simulink model "main_RI_LIEKF_GNSSOutrage"  (R2023a)
settings: Solver=FixedStepAuto  StartTime=0.0  StopTime=220  FixedStep=0.01  RelTol=1e-3
InitFcn:
  | initNavigation0612_AOA;
values from neighbouring files (symbols this model uses):
  CF_enable = 0    [initNavigation.m]
  dt = 0.01    [initNavigation.m]
  dtDelay = -0.03    [initNavigation.m]
  g0 = 9.795    [initNavigation.m]
  gam0_rad = 0/57.3    (= 0)    [initNavigation.m]
  GNSSoutragetime = 90    [initNavigation.m]
  H_sensor_type = 0    [initNavigation.m]
  KF_enable = 1    [initNavigation.m]
  P0 = diag([1*ones(3,1);0.01*ones(3,1);0.1*ones(3,1);0.001*ones(3,1);0.00001*ones(3,1)])    [initNavigation.m]
  P0_RIEKF = diag([1*ones(3,1);0.01*ones(3,1);0.1*ones(3,1);0.001*ones(3,1);0.00001*ones(3,1);      0.01*ones(3,1);[0;2;2]/57.3;[0.1;0.1;0.1]])^2    [initNavigation.m]
  pd0 = 0    [initNavigation.m]
  pe0 = 0    [initNavigation.m]
  phi0_rad = 0/57.3    (= 0)    [initNavigation.m]
  pn0 = 0    [initNavigation.m]
  psi = -178    [initNavigation.m]
  psi0_rad = 0/57.3    (= 0)    [initNavigation.m]
  state_dim = 24    [initNavigation.m]
  Time = 0:0.01:(size(traindata.AttackAngle,1) - 1)*0.01    [NNLiftCoefficientFit.m]
  vd0 = 0    [initNavigation.m]
  ve0 = 0    [initNavigation.m]
  vn0 = 0    [initNavigation.m]
undefined symbols (not defined in the file or in its folder): DiscIntNeverNeededParam, Discrete, INS_CONST, INS_EXPORT, INS_PARAM, magnitude, p, param, pInitialization, sys
libraries: simulink_extras x94, simulink x82, dspstat3 x70, sharedtransform x60, ctrlSharedLib x36, sharedTrackingLibrary x22, matrix_library x15, FMT_Model_Lib x13, deeplib x8, dspsolvers x4, vrlib x4, aerolibconvert2 x1
(part 3 of 28)

== system main_RI_LIEKF_GNSSOutrage/State estimation/15dim KF1/Error State Kalman Filter ==
  Sensor_data : Inport
  INS state : Inport  Port=2
  Add : Sum  Inputs=+-
  Bus Creator : BusCreator  Inputs=5
  Bus Selector : BusSelector  OutputSignals=QGC_sensor_reinit,GPS_Data.pos_N_gps,GPS_Data.pos_E_gps,GPS_Data.pos_D_gps,GPS_Data.vn_gps,GPS_Data.ve_gps,GPS_Data.vd_gps,vicon.vicon_posxyz,QGC_sensor_reinit
  Bus Selector2 : BusSelector  OutputSignals=RotationData.DCM_b_n,INSstate_v,INSstste_p,INSstate_w,INSstate_fb
  Cal Phi : Subsystem
  Cal Q : Subsystem
  Constant6 : Constant  Value=[eye(3),zeros(3,12)]  OutDataTypeStr=single
  Constant7 : Constant  Value=zeros(15,1)  OutDataTypeStr=single
  Data Store Read1 : DataStoreRead  DataStoreName=feedback_flag  IndexOptions=Index vector (dialog)  Indices=1  OutputSizes=1
  Data Store Read2 : DataStoreRead  DataStoreName=feedback_flag  IndexOptions=Index vector (dialog)  Indices=1  OutputSizes=1
  Data Type Conversion{1..3,5} (4 alike) : DataTypeConversion  OutDataTypeStr=single  SaturateOnIntegerOverflow=off  RndMeth=Floor
  Extract Diagonal : matrix_library/Extract Diagonal
  GNSS/INS Kalman Filter1 : Subsystem  AncestorBlock=ctrlSharedLib/Kalman Filter  mask(ctrlKalmanFilter){TimeDomain=Discrete-Time, UseCurrentEstimator=off, ModelSource=Input port, ModelSourceVariable=sys, A=0.95*eye(2), B=eye(2), C=eye(2), D=zeros(2), NumberOfStates=15, NumberOfInputs=0, NumberOfOutputs=3, InitialEstimateSource=Input port, X0=0, P0=10, UseK=off, UseGH=off, NumberOfProcessNoiseInputs=2, G=diag([zeros(3,1);ones(12,1)]), TimeInvariantG=off, H=0, TimeInvariantH=on, Q=diag([zeros(3,1);1e-2*ones(3,1);1e-4*ones(3,1);zeros(3,1);1e-5*ones(3,1)]), TimeInvariantQ=off, R=diag([0.001,0.001,0.001]), TimeInvariantR=on, N=0, TimeInvariantN=on, AddInputPort=off, AddEnablePort=on, ExternalReset=Rising, OutputEstimatedY=off, OutputP=on, Ts=dt}
      mask prompts: TimeDomain "Controllib:blocks:maskPromptKFTimeDomain"; UseCurrentEstimator "Controllib:blocks:maskPromptKFUseCurrentMeasurement"; ModelSource "Controllib:blocks:maskPromptKFModelSource"; ModelSourceVariable "Controllib:blocks:maskPromptKFModelSourceVariable"; A "Controllib:blocks:maskPromptKFA"; B "Controllib:blocks:maskPromptKFB"; C "Controllib:blocks:maskPromptKFC"; D "Controllib:blocks:maskPromptKFD"; NumberOfStates "Controllib:blocks:maskPromptKFNumberOfStates"; NumberOfInputs "Controllib:blocks:maskPromptKFNumberOfInputs"; NumberOfOutputs "Controllib:blocks:maskPromptKFNumberOfOutputs"; InitialEstimateSource "Controllib:blocks:maskPromptKFSource"; X0 "Controllib:blocks:maskPromptKFX0DT"; P0 "Controllib:blocks:maskPromptKFP0DT"; UseK "Controllib:blocks:maskPromptKFUseK"; UseGH "Controllib:blocks:maskPromptKFUseGH"; NumberOfProcessNoiseInputs "Controllib:blocks:maskPromptKFNumberOfProcessNoiseInputs"; G "Controllib:blocks:maskPromptKFG"; TimeInvariantG "Controllib:blocks:maskPromptKFTimeInvariantG"; H "Controllib:blocks:maskPromptKFH"; TimeInvariantH "Controllib:blocks:maskPromptKFTimeInvariantH"; Q "Controllib:blocks:maskPromptKFQ"; TimeInvariantQ "Controllib:blocks:maskPromptKFTimeInvariantQ"; R "Controllib:blocks:maskPromptKFR"; TimeInvariantR "Controllib:blocks:maskPromptKFTimeInvariantR"; N "Controllib:blocks:maskPromptKFN"; TimeInvariantN "Controllib:blocks:maskPromptKFTimeInvariantN"; AddInputPort "Controllib:blocks:maskPromptKFAddInputPort"; AddEnablePort "Controllib:blocks:maskPromptKFAddEnablePort"; ExternalReset "Simulink:blkprm_prompts:DelayBlkExternalReset"; OutputEstimatedY "Controllib:blocks:maskPromptKFOutputEstimatedY"; OutputP "Controllib:blocks:maskPromptKFOutputP"; Ts "Controllib:blocks:maskPromptKFTs"
      mask help: Controllib:blocks:maskPromptKFDescription
      mask init:
      | dlgParams.TimeDomain = TimeDomain;
      | dlgParams.UseCurrentEstimator = UseCurrentEstimator;
      | dlgParams.ModelSource = ModelSource;
      | dlgParams.ModelSourceVariable = ModelSourceVariable;
      | dlgParams.A = A;
      | dlgParams.B = B;
      | dlgParams.C = C;
      | dlgParams.D = D;
      | dlgParams.ModelHasFeedthrough = true();
      | dlgParams.NumberOfStates = NumberOfStates;
      | dlgParams.NumberOfInputs = NumberOfInputs;
      | dlgParams.NumberOfOutputs = NumberOfOutputs;
      | dlgParams.InitialEstimateSource = InitialEstimateSource;
      | dlgParams.X0 = X0;
      | dlgParams.P0 = P0;
      | dlgParams.UseGH = UseGH;
      | dlgParams.UseK = UseK;
      | dlgParams.NumberOfProcessNoiseInputs = NumberOfProcessNoiseInputs;
      | dlgParams.G = G;
      | dlgParams.TimeInvariantG = TimeInvariantG;
      | dlgParams.H = H;
      | dlgParams.TimeInvariantH = TimeInvariantH;
      | dlgParams.Q = Q;
      | dlgParams.TimeInvariantQ = TimeInvariantQ;
      | dlgParams.R = R;
      | dlgParams.TimeInvariantR = TimeInvariantR;
      | dlgParams.N = N;
      | dlgParams.TimeInvariantN = TimeInvariantN;
      | % Block options panel
      | dlgParams.OutputEstimatedY = OutputEstimatedY;
      | dlgParams.OutputP = OutputP;
      | dlgParams.AddEnablePort = AddEnablePort;
      | dlgParams.AddInputPort = AddInputPort;
      | dlgParams.ExternalReset = ExternalReset;
      | dlgParams.Ts = Ts;
      | [pInitialization,p] = ...
      |     controllib.internal.blocks.kalmanfilter.maskInitializationFcn(gcbh,dlgParams);
      | % Avoid storing dlg variables twice in the MaskWSVariables 
      | % block property
      | clear dlgParams;
      settings: LibrarySourceBlock=ctrlSharedLib/Kalman Filter
      mask Help: eval('controllib.internal.blocks.kalmanfilter.launchDocPage()')
      mask TypeOptions TimeDomain: Controllib:blocks:maskPromptKFTimeDomainDT | Controllib:blocks:maskPromptKFTimeDomainCT
      mask Callback TimeDomain: controllib.internal.blocks.kalmanfilter.dialogCallbacks(gcbh(),'comboBoxTimeDomain');
      mask Callback UseCurrentEstimator: controllib.internal.blocks.kalmanfilter.dialogCallbacks(gcbh(),'checkBoxUseCurrentEstimator');
      mask TypeOptions ModelSource: Controllib:blocks:maskPromptKFModelSourceLTIObject | Controllib:blocks:maskPromptKFModelSourceMatrices | Controllib:blocks:maskPromptKFSourceInport
      mask Callback ModelSource: controllib.internal.blocks.kalmanfilter.dialogCallbacks(gcbh(),'comboBoxModelSource');
      mask Callback ModelSourceVariable: controllib.internal.blocks.kalmanfilter.dialogCallbacks(gcbh(),'editBoxModelSourceVariable')
      mask TypeOptions InitialEstimateSource: Controllib:blocks:maskPromptKFSourceDialog | Controllib:blocks:maskPromptKFSourceInport
      mask Callback InitialEstimateSource: controllib.internal.blocks.kalmanfilter.dialogCallbacks(gcbh(),'comboBoxInitialEstimateSource');
      mask Callback UseK: controllib.internal.blocks.kalmanfilter.dialogCallbacks(gcbh(),'checkBoxUseK');
      mask Callback UseGH: controllib.internal.blocks.kalmanfilter.dialogCallbacks(gcbh(),'checkBoxUseGH');
      mask Callback TimeInvariantG: controllib.internal.blocks.kalmanfilter.dialogCallbacks(gcbh(),'checkBoxTimeInvariantGH');
      mask Callback TimeInvariantH: controllib.internal.blocks.kalmanfilter.dialogCallbacks(gcbh(),'checkBoxTimeInvariantGH');
      mask Callback TimeInvariantQ: controllib.internal.blocks.kalmanfilter.dialogCallbacks(gcbh(),'checkBoxTimeInvariantQRN');
      mask Callback TimeInvariantR: controllib.internal.blocks.kalmanfilter.dialogCallbacks(gcbh(),'checkBoxTimeInvariantQRN');
      mask Callback TimeInvariantN: controllib.internal.blocks.kalmanfilter.dialogCallbacks(gcbh(),'checkBoxTimeInvariantQRN');
      mask Callback AddInputPort: controllib.internal.blocks.kalmanfilter.dialogCallbacks(gcbh(),'checkBoxAddInputPort');
      mask TypeOptions ExternalReset: MemoryX/ExternalReset
      mask Callback OutputP: controllib.internal.blocks.kalmanfilter.dialogCallbacks(gcbh(),'checkBoxOutputP');
      mask DialogControl DescGroupVar Prompt: Controllib:blocks:maskPromptKFTitle
      mask DialogControl FilterSettingsContainer Prompt: Controllib:blocks:maskPromptKFContainerFilterSettings
      mask DialogControl TimeDomain Prompt: 时域:
      mask DialogControl UseCurrentEstimator Prompt: 使用当前测量 y[n] 来改进 xhat[n]
      mask DialogControl ModelParameterContainer Prompt: Controllib:blocks:maskPromptKFTabModelParameters
      mask DialogControl SystemModelContainer Prompt: Controllib:blocks:maskPromptKFContainerSystemModel
      mask DialogControl ModelSource Prompt: 模型源:
      mask DialogControl ModelSourceVariable Prompt: 变量:
      mask DialogControl A Prompt: A:
      mask DialogControl B Prompt: B:
      mask DialogControl C Prompt: C:
      mask DialogControl D Prompt: D:
      mask DialogControl NumberOfStates Prompt: 状态数量:
      mask DialogControl NumberOfInputs Prompt: 输入数目:
      mask DialogControl NumberOfOutputs Prompt: 输出数目:
      mask DialogControl InitialEstimatesContainer Prompt: Controllib:blocks:maskPromptKFContainerInitialEstimates
      mask DialogControl InitialEstimateSource Prompt: 源:
      mask DialogControl X0 Prompt: 初始状态 x[0]:
      mask DialogControl P0 Prompt: 状态估计误差协方差 P[0]
      mask DialogControl NoiseCharacteristicsContainer Prompt: Controllib:blocks:maskPromptKFContainerNoiseCharacteristics
      mask DialogControl UseK Prompt: 使用来自模型变量的 Kalman 增益 K
      mask DialogControl UseGH Prompt: 使用 G 和 H 矩阵(默认 G=I，H=0)
      mask DialogControl NumberOfProcessNoiseInputs Prompt: 过程噪声输入数目:
      mask DialogControl G Prompt: G:
      mask DialogControl TimeInvariantG Prompt: 时不变 G
      mask DialogControl H Prompt: H:
      mask DialogControl TimeInvariantH Prompt: 时不变 H
      mask DialogControl Q Prompt: Q:
      mask DialogControl TimeInvariantQ Prompt: 时不变 Q
      mask DialogControl R Prompt: R:
      mask DialogControl TimeInvariantR Prompt: 时不变 R
      mask DialogControl N Prompt: N:
      mask DialogControl TimeInvariantN Prompt: 时不变 N
      mask DialogControl OptionsContainer Prompt: Controllib:blocks:maskPromptKFTabOptions
      mask DialogControl AdditionalInportsContainer Prompt: Controllib:blocks:maskPromptKFContainerAdditionalInports
      mask DialogControl AddInputPort Prompt: 添加输入端口 u
      mask DialogControl AddEnablePort Prompt: 添加输入端口 Enable 以控制测量更新
      mask DialogControl ExternalReset Prompt: 外部重置:
      mask DialogControl AdditionalOutportsContainer Prompt: Controllib:blocks:maskPromptKFContainerAdditionalOutports
      mask DialogControl OutputEstimatedY Prompt: 输出估计的模型输出 y
      mask DialogControl OutputP Prompt: 输出状态估计误差协方差 P
      mask DialogControl Ts Prompt: 采样时间(-1 表示继承):
  Logical Operator : Logic  Commented=on  Operator=OR  AllPortsSameDT=off  OutDataTypeStr=boolean
  MATLAB Function : MATLAB Function  TreatAsAtomicUnit=on
  MATLAB Function2 : MATLAB Function  TreatAsAtomicUnit=on
  Memory : Memory
  Mux : Mux  Inputs=3
  Mux1 : Mux  Inputs=3
  Rate Transition : RateTransition  OutPortSampleTime=dt
  Rate Transition1 : RateTransition
  Rate Transition2 : RateTransition  OutPortSampleTime=dt
  Rate Transition3 : RateTransition  OutPortSampleTime=dt
  Scope{,2..3,5,7,9..10} (7 alike) : Scope
  Subsystem : Subsystem
  Terminator : Terminator
  delta_state : Outport
  Measuemrnt Enable Flag : Outport  Port=2
  covariance : Outport  Port=3
  wires:
  Data Store Read2/1 -> Logical Operator/1, GNSS/INS Kalman Filter1/5(Reset)
  Bus Selector/9 -> [QGC_init]  "<QGC_sensor_reinit>"
  Mux/1 -> [pos_NED]
  Rate Transition3/1 -> GNSS/INS Kalman Filter1/4(Enable)
  [Enable] -> Rate Transition3/1
  Memory/1 -> MATLAB Function/1(u)
  Bus Creator/1 -> delta_state/1
  MATLAB Function/3(dtheta) -> Bus Creator/3  "KFState_dtheta"
  Data Type Conversion1/1 -> Memory/1
  MATLAB Function/1(dp) -> Bus Creator/1  "KFState_dp"
  MATLAB Function/5(dg) -> Bus Creator/5  "KFState_da"
  MATLAB Function/2(dv) -> Bus Creator/2  "KFState_dv"
  MATLAB Function/4(da) -> Bus Creator/4  "KFState_da"
  Bus Selector2/3 -> [p_INS]  "<INSstste_p>"
  Bus Selector2/1 -> [DCM_b_n]  "<DCM_b_n>"
  Bus Selector2/5 -> [fbxyz]  "<INSstate_fb>"
  Bus Selector2/4 -> [wxyz]  "<INSstate_w>"
  INS state/1 -> Bus Selector2/1
  [Enable] -> Measuemrnt Enable Flag/1
  Bus Selector/4 -> Mux/3  "<pos_D_gps>"
  Bus Selector/2 -> Mux/1  "<pos_N_gps>"
  Bus Selector/3 -> Mux/2  "<pos_E_gps>"
  Bus Selector/7 -> Mux1/3  "<vd_gps>"
  Bus Selector/5 -> Mux1/1  "<vn_gps>"
  Mux1/1 -> Scope2/1, Terminator/1
  Sensor_data/1 -> Bus Selector/1
  Bus Selector/6 -> Mux1/2  "<ve_gps>"
  Extract Diagonal/1 -> Scope9/1, covariance/1
  GNSS/INS Kalman Filter1/2(P) -> Extract Diagonal/1
  Data Store Read1/1 -> Scope7/1
  Rate Transition2/1 -> Data Type Conversion5/1
  Cal Q/1(Qd) -> Rate Transition2/1
  MATLAB Function2/1(P) -> Data Type Conversion2/1
  Data Type Conversion5/1 -> GNSS/INS Kalman Filter1/8(Q)
  Cal Phi/1(Phi) -> Rate Transition1/1
  [DCM_b_n] -> Cal Phi/1(<DCM_b_n>)
  [pos_NED] -> Subsystem/1(data)
  [fbxyz] -> Cal Phi/3(axyz)
  Data Type Conversion2/1 -> GNSS/INS Kalman Filter1/3(P0)
  [pos_NED] -> Add/2, Scope3/1
  [p_INS] -> Add/1
  Rate Transition1/1 -> Data Type Conversion3/1
  [DCM_b_n] -> Cal Q/1(<DCM_b_n>)
  [wxyz] -> Cal Phi/2(wxyz)
  Add/1 -> Rate Transition/1, Scope10/1
  Data Type Conversion3/1 -> GNSS/INS Kalman Filter1/6(A)
  Constant6/1 -> GNSS/INS Kalman Filter1/7(C)
  [wxyz] -> Cal Q/2(wxyz)
  Rate Transition/1 -> GNSS/INS Kalman Filter1/1(y)
  Subsystem/1(flag) -> [Enable], Scope5/1
  GNSS/INS Kalman Filter1/1(xhat) -> Data Type Conversion1/1, Scope/1
  Constant7/1 -> GNSS/INS Kalman Filter1/2(X0)

== system main_RI_LIEKF_GNSSOutrage/State estimation/15dim KF1/INS propogation ==
  note: q(1:3)
  Sensor_data : Inport
  Measuemrnt Enable Flag : Inport  Port=2
  delta_state : Inport  Port=3
  Bus Creator : BusCreator  Inputs=7
  Bus Selector : BusSelector  OutputSignals=IMU_Data.gyro_B_rad/s_LPF,IMU_Data.accl_B_m/s2_LPF,MAGN_Data,QGC_sensor_reinit,GPS_Data.pos_N_gps,GPS_Data.pos_E_gps,GPS_Data.pos_D_gps,GPS_Data.vn_gps,GPS_Data.ve_gps,GPS_Data.vd_gps,vicon.vicon_posxyz
  Bus Selector1 : BusSelector  OutputSignals=DCM_b_n
  Bus Selector2 : BusSelector  OutputSignals=KFState_dp (signal 1),KFState_dv (signal 2),KFState_dtheta (signal 3),KFState_da (signal 4),KFState_da (signal 5)
  Data Type Conversion : DataTypeConversion  OutDataTypeStr=single  SaturateOnIntegerOverflow=off  RndMeth=Floor
  Init_PVQ2 : Subsystem
  Mux : Mux  Inputs=3
  Mux1 : Mux  Inputs=3
  accl bias compensation : Subsystem
  att_update : Subsystem
  gyro bias compensation : Subsystem
  vel_pos_update : Subsystem
  INSstate : Outport
  wires:
  Mux/1 -> [pos_NED]
  Bus Selector/2 -> [accl_raw]  "<accl_B_m/s2_LPF>"
  [accl_raw] -> accl bias compensation/1(raw <accl_B_m/s2_LPF>)
  [gyro_raw] -> gyro bias compensation/1(raw <gyro_B_rad/s_LPF>)
  Bus Selector2/5 -> [ddg]  "<KFState_da (signal 5)>"
  Bus Selector2/4 -> [dda]  "<KFState_da (signal 4)>"
  Bus Selector2/3 -> [dtheta]  "<KFState_dtheta (signal 3)>"
  Bus Selector2/2 -> [dv]  "<KFState_dv (signal 2)>"
  Bus Selector2/1 -> [dp]  "<KFState_dp (signal 1)>"
  delta_state/1 -> Bus Selector2/1
  [da] -> Bus Creator/7  "INSstate_da"
  [dg] -> Bus Creator/6  "INSstate_dg"
  gyro bias compensation/2(dg) -> [dg]
  gyro bias compensation/1(wb) -> [wxyz]
  Measuemrnt Enable Flag/1 -> gyro bias compensation/3(Measuemrnt Enable Flag)
  [ddg] -> gyro bias compensation/2(ddg)
  accl bias compensation/2(da) -> [da]
  accl bias compensation/1(fb) -> [fbxyz]
  [dda] -> accl bias compensation/2(dda)
  Bus Creator/1 -> INSstate/1
  att_update/1(att_update) -> Bus Creator/1, Bus Selector1/1  "RotationData"
  [fbxyz] -> Bus Creator/5  "INSstate_fb"
  [wxyz] -> Bus Creator/4  "INSstate_w"
  vel_pos_update/1(p_k) -> Bus Creator/2  "INSstste_p"
  [QGC_init] -> Init_PVQ2/1(QGC_sensor_reinit)
  [dv] -> vel_pos_update/7(dv)
  vel_pos_update/2(V) -> Bus Creator/3  "INSstate_v"
  Bus Selector1/1 -> vel_pos_update/1(<DCM_b_n>)  "<DCM_b_n>"
  Bus Selector/1 -> [gyro_raw]  "<gyro_B_rad/s_LPF>"
  Bus Selector/4 -> [QGC_init]  "<QGC_sensor_reinit>"
  [Magn] -> Init_PVQ2/3(Magn_B_guess_LPF)
  [dp] -> vel_pos_update/6(dp)
  Data Type Conversion/1 -> Init_PVQ2/5(vel_NED)
  [pos_NED] -> Init_PVQ2/4(pos_NED)
  [QGC_init] -> vel_pos_update/5(QGC_init)
  Bus Selector/9 -> Mux1/2  "<ve_gps>"
  Init_PVQ2/3(p0) -> vel_pos_update/4(p0)
  Init_PVQ2/2(v0) -> vel_pos_update/3(v0)
  [fbxyz] -> Init_PVQ2/2(accl_B_m/s2_LPF)
  Sensor_data/1 -> Bus Selector/1
  Mux1/1 -> [vel_NED]
  Bus Selector/3 -> [Magn]  "<MAGN_Data>"
  Bus Selector/6 -> Mux/2  "<pos_E_gps>"
  [wxyz] -> att_update/2(gyro)
  [dtheta] -> att_update/1(dtheta)
  Bus Selector/5 -> Mux/1  "<pos_N_gps>"
  Bus Selector/8 -> Mux1/1  "<vn_gps>"
  Bus Selector/7 -> Mux/3  "<pos_D_gps>"
  [vel_NED] -> Data Type Conversion/1
  Bus Selector/10 -> Mux1/3  "<vd_gps>"
  [QGC_init] -> att_update/4(init_flag)
  [fbxyz] -> vel_pos_update/2(Ab)
  Init_PVQ2/1(quat_0) -> att_update/3(quat_0)

== system main_RI_LIEKF_GNSSOutrage/State estimation/15dim KF1/Subsystem2 ==
  Z : Inport
  F : Inport  Port=2
  H : Inport  Port=3
  R : Inport  Port=4
  Q : Inport  Port=5
  P0 : Inport  Port=6
  X0 : Inport  Port=7
  enable : Inport  Port=8
  Constant : Constant  Value=zeros(15,1)
  Delay : Delay  DelayLength=1  InitialConditionSource=Input port
      settings: InputPortMap=u0,p4
  Delay1 : Delay  DelayLength=1  InitialConditionSource=Input port
      settings: InputPortMap=u0,p4
  Measurement Update : Subsystem
  NOT : Logic  Operator=NOT  IconShape=distinctive  AllPortsSameDT=off  OutDataTypeStr=boolean
  Reshape : Reshape  OutputDimensionality=Column vector (2-D)
  Reshape1 : Reshape  OutputDimensionality=Column vector (2-D)
  Switch : Switch  Criteria=u2 ~= 0  SaturateOnIntegerOverflow=off  InputSameDT=off
  Time Update : Subsystem
  enable1 : InportShadow  Port=8
  Xk : Outport
  Pk : Outport  Port=2
  wires:
  Z/1 -> Measurement Update/1(Z)
  Q/1 -> Time Update/2(Q)
  Time Update/1(Xk/k_1) -> Measurement Update/4(Xk_k_1)
  Time Update/2(Pk/k_1) -> Measurement Update/5(Pk_k_1)
  F/1 -> Time Update/1(F)
  H/1 -> Measurement Update/2(H)
  R/1 -> Measurement Update/3(R)
  Measurement Update/2(Pk) -> Pk/1, Delay1/1
  X0/1 -> Reshape1/1
  Delay/1 -> Time Update/4(X)
  P0/1 -> Delay1/2
  Delay1/1 -> Time Update/3(P)
  Reshape1/1 -> Delay/2
  Reshape/1 -> Xk/1
  enable/1 -> NOT/1
  NOT/1 -> Switch/2
  Constant/1 -> Switch/1
  Measurement Update/1(Xk) -> Switch/3
  Switch/1 -> Delay/1, Reshape/1
  enable1/1 -> Measurement Update/Enable

== system main_RI_LIEKF_GNSSOutrage/State estimation/Bus_Constructor1/Rotation_output ==
  RotationData : Inport
  Bus Creator : BusCreator  Inputs=3
  Bus Selector3 : BusSelector  OutputSignals=q_update
  Data Type Conversion11 : DataTypeConversion  OutDataTypeStr=single  SaturateOnIntegerOverflow=off  RndMeth=Floor
  Data Type Conversion12 : DataTypeConversion  OutDataTypeStr=double  SaturateOnIntegerOverflow=off  RndMeth=Floor
  Demux : Demux  Outputs=3
  JPL2Hem : MATLAB Function  TreatAsAtomicUnit=on
  Quaternions to Rotation Angles1 : sharedtransform/Quaternions to Rotation Angles  rotationOrder=ZYX  aMode=aMode
  Radians to Degrees : simulink_extras/Transformations/Radians to Degrees
  Signal Copy1 : SignalConversion  OverrideOpt=off
  psi_theta_phi_rad : Outport
  wires:
  Data Type Conversion12/1 -> JPL2Hem/1(q)
  RotationData/1 -> Signal Copy1/1
  Signal Copy1/1 -> Bus Selector3/1
  Bus Selector3/1 -> Data Type Conversion12/1  "<q_update>"
  Quaternions to Rotation Angles1/1 -> Radians to Degrees/1
  Bus Creator/1 -> psi_theta_phi_rad/1
  Demux/1 -> Bus Creator/1  "psi_rad"
  Demux/2 -> Bus Creator/2  "theta_rad"
  Demux/3 -> Bus Creator/3  "phi_rad"
  Data Type Conversion11/1 -> Demux/1
  JPL2Hem/1(y) -> Quaternions to Rotation Angles1/1
  Radians to Degrees/1 -> Data Type Conversion11/1

== system main_RI_LIEKF_GNSSOutrage/State estimation/Bus_Constructor2/Rotation_output ==
  RotationData : Inport
  Bus Creator : BusCreator  Inputs=3
  Bus Selector3 : BusSelector  OutputSignals=DCM_b_n
  Data Type Conversion11 : DataTypeConversion  OutDataTypeStr=single  SaturateOnIntegerOverflow=off  RndMeth=Floor
  Data Type Conversion12 : DataTypeConversion  OutDataTypeStr=double  SaturateOnIntegerOverflow=off  RndMeth=Floor
  Demux : Demux  Outputs=3
  Direction Cosine Matrix to Rotation Angles : sharedtransform/Direction Cosine Matrix to Rotation Angles  rotationOrder=ZYX  aMode=aMode  action=None  tolerance=eps(2)
      settings: LibrarySourceBlock=|
      | aerolibtransform2/Direction Cosine Matrix
      | to Rotation Angles
  Radians to Degrees : simulink_extras/Transformations/Radians to Degrees
  Signal Copy1 : SignalConversion  OverrideOpt=off
  Transpose : Math  Operator=transpose
  psi_theta_phi_rad : Outport
  wires:
  Data Type Conversion11/1 -> Demux/1
  Demux/3 -> Bus Creator/3  "phi_rad"
  Demux/2 -> Bus Creator/2  "theta_rad"
  Demux/1 -> Bus Creator/1  "psi_rad"
  Bus Creator/1 -> psi_theta_phi_rad/1
  Direction Cosine Matrix to Rotation Angles/1 -> Radians to Degrees/1
  Bus Selector3/1 -> Transpose/1  "<DCM_b_n>"
  Signal Copy1/1 -> Bus Selector3/1
  RotationData/1 -> Signal Copy1/1
  Data Type Conversion12/1 -> Direction Cosine Matrix to Rotation Angles/1
  Transpose/1 -> Data Type Conversion12/1
  Radians to Degrees/1 -> Data Type Conversion11/1

== system main_RI_LIEKF_GNSSOutrage/State estimation/Bus_Constructor3/Rotation_output ==
  RotationData : Inport
  Bus Creator : BusCreator  Inputs=3
  Bus Selector3 : BusSelector  OutputSignals=DCM_b_n
  Data Type Conversion11 : DataTypeConversion  OutDataTypeStr=single  SaturateOnIntegerOverflow=off  RndMeth=Floor
  Data Type Conversion12 : DataTypeConversion  OutDataTypeStr=double  SaturateOnIntegerOverflow=off  RndMeth=Floor
  Demux : Demux  Outputs=3
  Direction Cosine Matrix to Rotation Angles : sharedtransform/Direction Cosine Matrix to Rotation Angles  rotationOrder=ZYX  aMode=aMode  action=None  tolerance=eps(2)
      settings: LibrarySourceBlock=|
      | aerolibtransform2/Direction Cosine Matrix
      | to Rotation Angles
  Radians to Degrees : simulink_extras/Transformations/Radians to Degrees
  Signal Copy1 : SignalConversion  OverrideOpt=off
  Transpose : Math  Operator=transpose
  psi_theta_phi_rad : Outport
  wires:
  Radians to Degrees/1 -> Data Type Conversion11/1
  Transpose/1 -> Data Type Conversion12/1
  Data Type Conversion12/1 -> Direction Cosine Matrix to Rotation Angles/1
  RotationData/1 -> Signal Copy1/1
  Signal Copy1/1 -> Bus Selector3/1
  Bus Selector3/1 -> Transpose/1  "<DCM_b_n>"
  Direction Cosine Matrix to Rotation Angles/1 -> Radians to Degrees/1
  Bus Creator/1 -> psi_theta_phi_rad/1
  Demux/1 -> Bus Creator/1  "psi_rad"
  Demux/2 -> Bus Creator/2  "theta_rad"
  Demux/3 -> Bus Creator/3  "phi_rad"
  Data Type Conversion11/1 -> Demux/1

== system main_RI_LIEKF_GNSSOutrage/State estimation/ER EKF/Bus_Constructor ==
  INSstate : Inport
  Bus Creator : BusCreator  Inputs=2
  Bus Creator1 : BusCreator  Inputs=2
  Bus Creator3 : BusCreator  Inputs=6
  Bus Selector : BusSelector  OutputSignals=RotationData.q_update,RotationData.DCM_b_n,INSstate_v,INSstste_p,INSstate_dg,INSstate_da,INSstate_pL
  Demux2 : Demux  Outputs=3
  Demux3 : Demux  Outputs=3
  TranslationData : Outport
  RotationData : Outport  Port=2
  INSbiasData : Outport  Port=3
  wires:
  INSstate/1 -> Bus Selector/1
  Bus Selector/2 -> Bus Creator/2  "<DCM_b_n>"
  Bus Selector/1 -> Bus Creator/1  "<q_update>"
  Bus Creator/1 -> RotationData/1
  Bus Selector/5 -> Bus Creator1/1  "<INSstate_dg>"
  Bus Selector/6 -> Bus Creator1/2  "<INSstate_da>"
  Bus Creator1/1 -> INSbiasData/1
  Demux2/3 -> Bus Creator3/3  "vd_m/s"
  Demux2/1 -> Bus Creator3/1  "vn_m/s"
  Demux3/3 -> Bus Creator3/6  "pd_m"
  Demux3/1 -> Bus Creator3/4  "pn_m"
  Bus Creator3/1 -> TranslationData/1
  Demux2/2 -> Bus Creator3/2  "ve_m/s"
  Demux3/2 -> Bus Creator3/5  "pe_m"
  Bus Selector/3 -> Demux2/1  "<INSstate_v>"
  Bus Selector/4 -> Demux3/1  "<INSstste_p>"

== system main_RI_LIEKF_GNSSOutrage/State estimation/ER EKF/Error State Kalman Filter ==
  Sensor_data : Inport
  INS state : Inport  Port=2
  Add1 : Sum  Inputs=+-
  Add2 : Sum  Inputs=+-
  Bus Creator : BusCreator  Inputs=5
  Bus Creator1 : BusCreator  Inputs=2
  Bus Selector : BusSelector  OutputSignals=QGC_sensor_reinit,GPS_Data.pos_N_gps,GPS_Data.pos_E_gps,GPS_Data.pos_D_gps,GPS_Data.vn_gps,GPS_Data.ve_gps,GPS_Data.vd_gps
  Bus Selector2 : BusSelector  OutputSignals=RotationData.DCM_b_n,INSstate_v,INSstste_p,INSstate_w,INSstate_fb,INSstate_pL,INSstate_vL
  Cal Q1 : Subsystem
  Constant1 : Constant  Value=diag([0.001,0.001,0.001,0.0001,0.0001,0.0001])  OutDataTypeStr=single
  Data Store Read1 : DataStoreRead  DataStoreName=feedback_flag_18dim  IndexOptions=Index vector (dialog)  Indices=1  OutputSizes=1
  Data Store Read3 : DataStoreRead  DataStoreName=GPS_enable  IndexOptions=Index vector (dialog)  Indices=1  OutputSizes=1
  Data Store Read4 : DataStoreRead  DataStoreName=GPS_enable  IndexOptions=Index vector (dialog)  Indices=1  OutputSizes=1
  Data Store Read5 : DataStoreRead  DataStoreName=GPS_enable  IndexOptions=Index vector (dialog)  Indices=1  OutputSizes=1
  Data Store Read6 : DataStoreRead  DataStoreName=feedback_flag_18dim  IndexOptions=Index vector (dialog)  Indices=1  OutputSizes=1
  Data Store Write : DataStoreWrite  DataStoreName=GPS_enable  IndexOptions=Index vector (dialog)  Indices=1  OutputSizes=1
  Data Type Conversion1 : DataTypeConversion  OutDataTypeStr=single  SaturateOnIntegerOverflow=off  RndMeth=Floor
  Data Type Conversion6 : DataTypeConversion  OutDataTypeStr=single  SaturateOnIntegerOverflow=off  RndMeth=Floor
  Extended Kalman Filter1 : Subsystem  mask(Extended Kalman Filter){StateTransitionFcn=stateTransitionFcn, HasStateTransitionJacobianFcn=on, StateTransitionJacobianFcn=stateTransitionJacobianFcn, HasAdditiveProcessNoise=Nonadditive, ProcessNoise=1, HasTimeVaryingProcessNoise=on, HasStateTransitionFcnExtraArgument=0, InitialState=zeros(15,1), InitialStateCovariance=P0, MeasurementFcn1=GPSMeasurementFcn, HasMeasurementJacobianFcn1=off, MeasurementJacobianFcn1=, HasMeasurementEnablePort1=on, HasAdditiveMeasurementNoise1=Nonadditive, MeasurementNoise1=1, HasTimeVaryingMeasurementNoise1=on, HasMeasurementFcnExtraArgument1=0, HasMeasurementWrapping1=off, MeasurementFcn2=DynamicMeasurementFcn_Dyn, HasMeasurementJacobianFcn2=off, MeasurementJacobianFcn2=, HasMeasurementEnablePort2=on, HasAdditiveMeasurementNoise2=Nonadditive, MeasurementNoise2=1, HasTimeVaryingMeasurementNoise2=on, HasMeasurementFcnExtraArgument2=0, HasMeasurementWrapping2=off, MeasurementFcn3=ZUPTMeasurementFcn2, HasMeasurementJacobianFcn3=off, MeasurementJacobianFcn3=, HasMeasurementEnablePort3=on, HasAdditiveMeasurementNoise3=Nonadditive, MeasurementNoise3=1, HasTimeVaryingMeasurementNoise3=on, HasMeasurementFcnExtraArgument3=0, HasMeasurementWrapping3=off, MeasurementFcn4=myMeasurementFcn, HasMeasurementJacobianFcn4=off, MeasurementJacobianFcn4=, HasMeasurementEnablePort4=off, HasAdditiveMeasurementNoise4=Additive, MeasurementNoise4=1, HasTimeVaryingMeasurementNoise4=off, HasMeasurementFcnExtraArgument4=0, HasMeasurementWrapping4=off, MeasurementFcn5=myMeasurementFcn, HasMeasurementJacobianFcn5=off, MeasurementJacobianFcn5=, HasMeasurementEnablePort5=off, HasAdditiveMeasurementNoise5=Additive, MeasurementNoise5=1, HasTimeVaryingMeasurementNoise5=off, HasMeasurementFcnExtraArgument5=0, HasMeasurementWrapping5=off, EnableMultirate=off, StateTransitionFcnSampleTime=0.01, MeasurementFcn1SampleTime=0.2, MeasurementFcn2SampleTime=0.01, MeasurementFcn3SampleTime=1, MeasurementFcn4SampleTime=1, MeasurementFcn5SampleTime=1, UseCurrentEstimator=on, OutputStateCovariance=on, DataType=single, SampleTime=0.01, NumberOfMeasurements=1}
      mask prompts: HasStateTransitionJacobianFcn "shared_tracking:blocks:maskPromptEKFJacobian"; HasTimeVaryingProcessNoise "shared_tracking:blocks:maskPromptEKFUKFTimeVarying"; HasMeasurementJacobianFcn1 "shared_tracking:blocks:maskPromptEKFJacobian"; HasMeasurementEnablePort1 "shared_tracking:blocks:maskPromptEnablePort"; HasTimeVaryingMeasurementNoise1 "shared_tracking:blocks:maskPromptEKFUKFTimeVarying"; HasMeasurementWrapping1 "shared_tracking:blocks:maskPromptEKFUKFMeasurementWrapping"; HasMeasurementJacobianFcn2 "shared_tracking:blocks:maskPromptEKFJacobian"; HasMeasurementEnablePort2 "shared_tracking:blocks:maskPromptEnablePort"; HasTimeVaryingMeasurementNoise2 "shared_tracking:blocks:maskPromptEKFUKFTimeVarying"; HasMeasurementWrapping2 "shared_tracking:blocks:maskPromptEKFUKFMeasurementWrapping"; HasMeasurementJacobianFcn3 "shared_tracking:blocks:maskPromptEKFJacobian"; HasMeasurementEnablePort3 "shared_tracking:blocks:maskPromptEnablePort"; HasTimeVaryingMeasurementNoise3 "shared_tracking:blocks:maskPromptEKFUKFTimeVarying"; HasMeasurementWrapping3 "shared_tracking:blocks:maskPromptEKFUKFMeasurementWrapping"; HasMeasurementJacobianFcn4 "shared_tracking:blocks:maskPromptEKFJacobian"; HasMeasurementEnablePort4 "shared_tracking:blocks:maskPromptEnablePort"; HasTimeVaryingMeasurementNoise4 "shared_tracking:blocks:maskPromptEKFUKFTimeVarying"; HasMeasurementWrapping4 "shared_tracking:blocks:maskPromptEKFUKFMeasurementWrapping"; HasMeasurementJacobianFcn5 "shared_tracking:blocks:maskPromptEKFJacobian"; HasMeasurementEnablePort5 "shared_tracking:blocks:maskPromptEnablePort"; HasTimeVaryingMeasurementNoise5 "shared_tracking:blocks:maskPromptEKFUKFTimeVarying"; HasMeasurementWrapping5 "shared_tracking:blocks:maskPromptEKFUKFMeasurementWrapping"; EnableMultirate "shared_tracking:blocks:maskPromptEnableMultirate"; StateTransitionFcnSampleTime "shared_tracking:blocks:maskPromptStateTransition"; MeasurementFcn1SampleTime "shared_tracking:blocks:maskPromptMeasurement1"; MeasurementFcn2SampleTime "shared_tracking:blocks:maskPromptMeasurement2"; MeasurementFcn3SampleTime "shared_tracking:blocks:maskPromptMeasurement3"; MeasurementFcn4SampleTime "shared_tracking:blocks:maskPromptMeasurement4"; MeasurementFcn5SampleTime "shared_tracking:blocks:maskPromptMeasurement5"; UseCurrentEstimator "shared_tracking:blocks:maskPromptUseCurrentEstimator"; OutputStateCovariance "shared_tracking:blocks:maskPromptOutputStateCovariance"; DataType "shared_tracking:blocks:maskPromptDataType"; SampleTime "shared_tracking:blocks:maskPromptSampleTime"
      mask help: shared_tracking:blocks:maskPromptEKFDescription
      mask init:
      | matlabshared.tracking.internal.blocks.maskInitializationScriptEKF
      mask Help: eval('matlabshared.tracking.internal.blocks.controlIdentLaunchDocPage(''EKF'')')
      mask Callback HasStateTransitionJacobianFcn: matlabshared.tracking.internal.blocks.dialogCallbacksEKFUKFPF(gcbh(),'checkBoxHasJacobianFcn','StateTransition');
      mask TypeOptions HasAdditiveProcessNoise: shared_tracking:blocks:maskPromptEKFUKFAdditiveNoise | shared_tracking:blocks:maskPromptEKFUKFNonAdditiveNoise
      mask Callback HasTimeVaryingProcessNoise: matlabshared.tracking.internal.blocks.dialogCallbacksEKFUKFPF(gcbh,'checkboxIsCovarianceTimeVarying','HasTimeVaryingProcessNoise','ProcessNoise')
      mask Callback HasMeasurementJacobianFcn1: matlabshared.tracking.internal.blocks.dialogCallbacksEKFUKFPF(gcbh(),'checkBoxHasJacobianFcn','Measurement','1');
      mask TypeOptions HasAdditiveMeasurementNoise1: shared_tracking:blocks:maskPromptEKFUKFAdditiveNoise | shared_tracking:blocks:maskPromptEKFUKFNonAdditiveNoise
      mask Callback HasTimeVaryingMeasurementNoise1: matlabshared.tracking.internal.blocks.dialogCallbacksEKFUKFPF(gcbh,'checkboxIsCovarianceTimeVarying','HasTimeVaryingMeasurementNoise1','MeasurementNoise1')
      mask Callback HasMeasurementJacobianFcn2: matlabshared.tracking.internal.blocks.dialogCallbacksEKFUKFPF(gcbh(),'checkBoxHasJacobianFcn','Measurement','2');
      mask TypeOptions HasAdditiveMeasurementNoise2: shared_tracking:blocks:maskPromptEKFUKFAdditiveNoise | shared_tracking:blocks:maskPromptEKFUKFNonAdditiveNoise
      mask Callback HasTimeVaryingMeasurementNoise2: matlabshared.tracking.internal.blocks.dialogCallbacksEKFUKFPF(gcbh,'checkboxIsCovarianceTimeVarying','HasTimeVaryingMeasurementNoise2','MeasurementNoise2')
      mask Callback HasMeasurementJacobianFcn3: matlabshared.tracking.internal.blocks.dialogCallbacksEKFUKFPF(gcbh(),'checkBoxHasJacobianFcn','Measurement','3');
      mask TypeOptions HasAdditiveMeasurementNoise3: shared_tracking:blocks:maskPromptEKFUKFAdditiveNoise | shared_tracking:blocks:maskPromptEKFUKFNonAdditiveNoise
      mask Callback HasTimeVaryingMeasurementNoise3: matlabshared.tracking.internal.blocks.dialogCallbacksEKFUKFPF(gcbh,'checkboxIsCovarianceTimeVarying','HasTimeVaryingMeasurementNoise3','MeasurementNoise3')
      mask Callback HasMeasurementJacobianFcn4: matlabshared.tracking.internal.blocks.dialogCallbacksEKFUKFPF(gcbh(),'checkBoxHasJacobianFcn','Measurement','4');
      mask TypeOptions HasAdditiveMeasurementNoise4: shared_tracking:blocks:maskPromptEKFUKFAdditiveNoise | shared_tracking:blocks:maskPromptEKFUKFNonAdditiveNoise
      mask Callback HasTimeVaryingMeasurementNoise4: matlabshared.tracking.internal.blocks.dialogCallbacksEKFUKFPF(gcbh,'checkboxIsCovarianceTimeVarying','HasTimeVaryingMeasurementNoise4','MeasurementNoise4')
      mask Callback HasMeasurementJacobianFcn5: matlabshared.tracking.internal.blocks.dialogCallbacksEKFUKFPF(gcbh(),'checkBoxHasJacobianFcn','Measurement','5');
      mask TypeOptions HasAdditiveMeasurementNoise5: shared_tracking:blocks:maskPromptEKFUKFAdditiveNoise | shared_tracking:blocks:maskPromptEKFUKFNonAdditiveNoise
      mask Callback HasTimeVaryingMeasurementNoise5: matlabshared.tracking.internal.blocks.dialogCallbacksEKFUKFPF(gcbh,'checkboxIsCovarianceTimeVarying','HasTimeVaryingMeasurementNoise5','MeasurementNoise5')
      mask Callback EnableMultirate: matlabshared.tracking.internal.blocks.dialogCallbacksEKFUKFPF(gcbh,'checkBoxHasMultirate')
      mask TypeOptions DataType: shared_tracking:blocks:maskPromptDouble | shared_tracking:blocks:maskPromptSingle
      mask Callback NumberOfMeasurements: matlabshared.tracking.internal.blocks.dialogCallbacksEKFUKFPF(gcbh,'editboxNumberOfMeasurements','MeasurementFcn');
      mask DialogControl DescGroupVar Prompt: shared_tracking:blocks:maskPromptEKFTitle
      mask DialogControl TabSystemModel Prompt: shared_tracking:blocks:maskPromptSystemModel
      mask DialogControl GroupStateTransition Prompt: shared_tracking:blocks:maskPromptStateTransition
      mask DialogControl StateTransitionFunctionText Prompt: shared_tracking:blocks:maskPromptFunction
      mask DialogControl HasStateTransitionJacobianFcn Prompt: Jacobian
      mask DialogControl ProcessNoiseText Prompt: shared_tracking:blocks:maskPromptEKFUKFProcessNoise
      mask DialogControl ProcessNoiseCovarianceText Prompt: shared_tracking:blocks:maskPromptCovariance
      mask DialogControl HasTimeVaryingProcessNoise Prompt: Time-varying
      mask DialogControl InitializationContainer Prompt: shared_tracking:blocks:maskPromptInitialization
      mask DialogControl InitialStateText Prompt: shared_tracking:blocks:maskPromptEKFUKFInitialState
      mask DialogControl InitialCovarianceText Prompt: shared_tracking:blocks:maskPromptEKFUKFInitialCovariance
      mask DialogControl GroupMeasurement1 Prompt: shared_tracking:blocks:maskPromptMeasurement1
      mask DialogControl MeasurementFunction1Text Prompt: shared_tracking:blocks:maskPromptFunction
      mask DialogControl HasMeasurementJacobianFcn1 Prompt: Jacobian
      mask DialogControl HasMeasurementEnablePort1 Prompt: Add Enable port
      mask DialogControl MeasurementNoiseText1 Prompt: shared_tracking:blocks:maskPromptEKFUKFMeasurementNoise
      mask DialogControl MeasurementNoiseCovarianceText1 Prompt: shared_tracking:blocks:maskPromptCovariance
      mask DialogControl HasTimeVaryingMeasurementNoise1 Prompt: Time-varying
      mask DialogControl HasMeasurementWrapping1 Prompt: Has measurement wrapping
      mask DialogControl GroupMeasurement2 Prompt: shared_tracking:blocks:maskPromptMeasurement2
      mask DialogControl MeasurementFunction2Text Prompt: shared_tracking:blocks:maskPromptFunction
      mask DialogControl HasMeasurementJacobianFcn2 Prompt: Jacobian
      mask DialogControl HasMeasurementEnablePort2 Prompt: Add Enable port
      mask DialogControl MeasurementNoiseText2 Prompt: shared_tracking:blocks:maskPromptEKFUKFMeasurementNoise
      mask DialogControl MeasurementNoiseCovarianceText2 Prompt: shared_tracking:blocks:maskPromptCovariance
      mask DialogControl HasTimeVaryingMeasurementNoise2 Prompt: Time-varying
      mask DialogControl HasMeasurementWrapping2 Prompt: Has measurement wrapping
      mask DialogControl GroupMeasurement3 Prompt: shared_tracking:blocks:maskPromptMeasurement3
      mask DialogControl MeasurementFunction3Text Prompt: shared_tracking:blocks:maskPromptFunction
      mask DialogControl HasMeasurementJacobianFcn3 Prompt: Jacobian
      mask DialogControl HasMeasurementEnablePort3 Prompt: Add Enable port
      mask DialogControl MeasurementNoiseText3 Prompt: shared_tracking:blocks:maskPromptEKFUKFMeasurementNoise
      mask DialogControl MeasurementNoiseCovarianceText3 Prompt: shared_tracking:blocks:maskPromptCovariance
      mask DialogControl HasTimeVaryingMeasurementNoise3 Prompt: Time-varying
      mask DialogControl HasMeasurementWrapping3 Prompt: Has measurement wrapping
      mask DialogControl GroupMeasurement4 Prompt: shared_tracking:blocks:maskPromptMeasurement4
      mask DialogControl MeasurementFunction4Text Prompt: shared_tracking:blocks:maskPromptFunction
      mask DialogControl HasMeasurementJacobianFcn4 Prompt: Jacobian
      mask DialogControl HasMeasurementEnablePort4 Prompt: Add Enable port
      mask DialogControl MeasurementNoiseText4 Prompt: shared_tracking:blocks:maskPromptEKFUKFMeasurementNoise
      mask DialogControl MeasurementNoiseCovarianceText4 Prompt: shared_tracking:blocks:maskPromptCovariance
      mask DialogControl HasTimeVaryingMeasurementNoise4 Prompt: Time-varying
      mask DialogControl HasMeasurementWrapping4 Prompt: Has measurement wrapping
      mask DialogControl GroupMeasurement5 Prompt: shared_tracking:blocks:maskPromptMeasurement5
      mask DialogControl MeasurementFunction5Text Prompt: shared_tracking:blocks:maskPromptFunction
      mask DialogControl HasMeasurementJacobianFcn5 Prompt: Jacobian
      mask DialogControl HasMeasurementEnablePort5 Prompt: Add Enable port
      mask DialogControl MeasurementNoiseText5 Prompt: shared_tracking:blocks:maskPromptEKFUKFMeasurementNoise
      mask DialogControl MeasurementNoiseCovarianceText5 Prompt: shared_tracking:blocks:maskPromptCovariance
      mask DialogControl HasTimeVaryingMeasurementNoise5 Prompt: Time-varying
      mask DialogControl HasMeasurementWrapping5 Prompt: Has measurement wrapping
      mask DialogControl AddMeasurement Prompt: shared_tracking:blocks:maskPromptAddMeasurement
      mask DialogControl AddMeasurement Callback: matlabshared.tracking.internal.blocks.dialogCallbacksEKFUKFPF(gcbh,'buttonAddMeasurement','MeasurementFcn');
      mask DialogControl RemoveMeasurement Prompt: shared_tracking:blocks:maskPromptRemoveMeasurement
      mask DialogControl RemoveMeasurement Callback: matlabshared.tracking.internal.blocks.dialogCallbacksEKFUKFPF(gcbh,'buttonRemoveMeasurement','MeasurementFcn');
      mask DialogControl TabMultirate Prompt: shared_tracking:blocks:maskPromptEKFUKFMultirate
      mask DialogControl GroupMultirate Prompt: shared_tracking:blocks:maskPromptEKFUKFMultirate
      mask DialogControl EnableMultirate Prompt: Enable multirate operation
      mask DialogControl GroupMultirateSampleTimes Prompt: shared_tracking:blocks:maskPromptSampleTimeNoInheritance
      mask DialogControl StateTransitionFcnSampleTime Prompt: State Transition
      mask DialogControl MeasurementFcn1SampleTime Prompt: Measurement 1
      mask DialogControl MeasurementFcn2SampleTime Prompt: Measurement 2
      mask DialogControl MeasurementFcn3SampleTime Prompt: Measurement 3
      mask DialogControl MeasurementFcn4SampleTime Prompt: Measurement 4
      mask DialogControl MeasurementFcn5SampleTime Prompt: Measurement 5
      mask DialogControl ContainerSettings Prompt: shared_tracking:blocks:maskPromptEKFUKFSettings
      mask DialogControl UseCurrentEstimator Prompt: Use the current measurements to improve state estimates
      mask DialogControl OutputStateCovariance Prompt: Output state estimation error covariance
      mask DialogControl DataType Prompt: Data type:
      mask DialogControl SampleTime Prompt: Sample time:
  Extract Diagonal1 : matrix_library/Extract Diagonal
  From2 : From  Commented=on  GotoTag=wxyz
  From3 : From  Commented=on  GotoTag=fbxyz
  From5 : From  Commented=on  GotoTag=fex
  From6 : From  Commented=on  GotoTag=DCM_b_n
  Goto6 : Goto  Commented=on  GotoTag=ZUPTenable
  Logical Operator : Logic  AllPortsSameDT=off  OutDataTypeStr=boolean
  MATLAB Function : MATLAB Function  TreatAsAtomicUnit=on
  MATLAB Function1 : MATLAB Function  Commented=on  TreatAsAtomicUnit=on
  Memory : Memory
  Memory1 : Memory  Commented=on
  Mux : Mux  Inputs=3
  Mux1 : Mux  Inputs=3
  Mux2 : Mux  Inputs=2
  Rate Transition{5..8} (4 alike) : RateTransition  OutPortSampleTime=dt
  Scope{,1..3,5..7} (7 alike) : Scope
  Scope10 : Scope  Commented=on  NumInputPorts=2
  Scope8 : Scope  NumInputPorts=2
  Simulink Function - GPS Measurements : Subsystem  TreatAsAtomicUnit=on
  Simulink Function - GPS Measurements1 : Subsystem  TreatAsAtomicUnit=on
  Simulink Function - GPS Measurements2 : Subsystem  TreatAsAtomicUnit=on
  Simulink Function - State Transition : Subsystem  TreatAsAtomicUnit=on
  Simulink Function - State Transition Jacobian : Subsystem  TreatAsAtomicUnit=on
  Step : Step  Time=GNSSoutragetime  Before=1  After=0  SampleTime=0
  Subsystem : Subsystem
  Terminator : Terminator
  delta_state : Outport
  Measuemrnt Enable Flag : Outport  Port=2
  EKFState : Outport  Port=3
  wires:
  Mux/1 -> Scope3/1, [pos_NED]
  Data Store Read6/1 -> Scope8/2
  Data Store Read5/1 -> Scope8/1
  Data Type Conversion6/1 -> Extended Kalman Filter1/1(Q)
  Rate Transition5/1 -> Data Type Conversion6/1
  Cal Q1/1(Qd) -> Rate Transition5/1
  Rate Transition8/1 -> Extended Kalman Filter1/4(R1)
  Rate Transition7/1 -> Extended Kalman Filter1/3(y1)
  Rate Transition6/1 -> Extended Kalman Filter1/2(Enable1)
  Extract Diagonal1/1 -> Scope6/1, Bus Creator1/2  "covariance"
  Extended Kalman Filter1/2(P) -> Extract Diagonal1/1
  Mux2/1 -> Scope1/1, Rate Transition7/1
  [pos_NED] -> Add1/2
  [p_INS] -> Add1/1
  Constant1/1 -> Rate Transition8/1
  [DCM_b_n] -> Simulink Function - GPS Measurements1/1(DCM_b_n)
  [fbxyz] -> Simulink Function - State Transition Jacobian/3(fbxyz)
  [fbxyz] -> Simulink Function - State Transition/3(fbxyz)
  [wxyz] -> Simulink Function - State Transition Jacobian/2(wxyz)
  [wxyz] -> Simulink Function - State Transition/2(wxyz)
  [DCM_b_n] -> Simulink Function - State Transition Jacobian/1(DCM_b_n)
  [DCM_b_n] -> Simulink Function - State Transition/1(DCM_b_n)
  MATLAB Function/3(dtheta) -> Bus Creator/3  "KFState_dtheta"
  MATLAB Function/1(dp) -> Bus Creator/1  "KFState_dp"
  Extended Kalman Filter1/1(xhat) -> Data Type Conversion1/1, Scope/1
  Subsystem/1(flag) -> Scope5/1, Data Store Write/1
  [pos_NED] -> Subsystem/1(data)
  Data Store Read1/1 -> Scope7/1
  Bus Selector/6 -> Mux1/2  "<ve_gps>"
  Sensor_data/1 -> Bus Selector/1
  Mux1/1 -> Terminator/1, Scope2/1, [vel_NED]
  Bus Selector/5 -> Mux1/1  "<vn_gps>"
  Bus Selector/7 -> Mux1/3  "<vd_gps>"
  Bus Selector/3 -> Mux/2  "<pos_E_gps>"
  Bus Selector/2 -> Mux/1  "<pos_N_gps>"
  Bus Selector/4 -> Mux/3  "<pos_D_gps>"
  Data Store Read4/1 -> Measuemrnt Enable Flag/1
  INS state/1 -> Bus Selector2/1
  Bus Selector2/4 -> [wxyz]  "<INSstate_w>"
  Bus Selector2/5 -> [fbxyz]  "<INSstate_fb>"
  Bus Selector2/1 -> [DCM_b_n]  "<DCM_b_n>"
  MATLAB Function/4(da) -> Bus Creator/4  "KFState_da"
  MATLAB Function/2(dv) -> Bus Creator/2  "KFState_dv"
  MATLAB Function/5(dg) -> Bus Creator/5  "KFState_dg"
  Data Type Conversion1/1 -> Memory/1
  Bus Creator/1 -> Bus Creator1/1, delta_state/1  "delta_state"
  Memory/1 -> MATLAB Function/1(u)
  Add1/1 -> Mux2/1
  Add2/1 -> Mux2/2
  [v_INS] -> Add2/1
  [vel_NED] -> Add2/2
  From6/1 -> MATLAB Function1/1(Cbn)
  From3/1 -> MATLAB Function1/3(fbxyz)
  MATLAB Function1/2(ZeroVelDetectFlagold) -> Scope10/2
  Memory1/1 -> MATLAB Function1/4(fex)
  From5/1 -> Memory1/1
  From2/1 -> MATLAB Function1/2(wxyz)
  MATLAB Function1/1(ZeroVelDetectFlag) -> Scope10/1, Goto6/1
  Bus Creator1/1 -> EKFState/1
  Bus Selector2/6 -> [p_INS]  "<INSstate_pL>"
  Bus Selector2/7 -> [v_INS]  "<INSstate_vL>"
  Step/1 -> Logical Operator/1
  Data Store Read3/1 -> Logical Operator/2
  Logical Operator/1 -> Rate Transition6/1
